simulink model "s0505_rollsensorfusion_EKF"  (R2021a)
settings: Solver=FixedStepAuto  StartTime=0.0  StopTime=10.0  RelTol=1e-3  EnableMultiTasking=on
undefined symbols (not defined in the file): Ts
libraries: CarMaker4SL x13, dspfdesign x2, dspmathops x2, sharedTrackingLibrary x1
settings Model: Creator=jason  LastModifiedBy=jason
settings ModelReferenceCC: ModelReferenceNumInstancesAllowed=Single

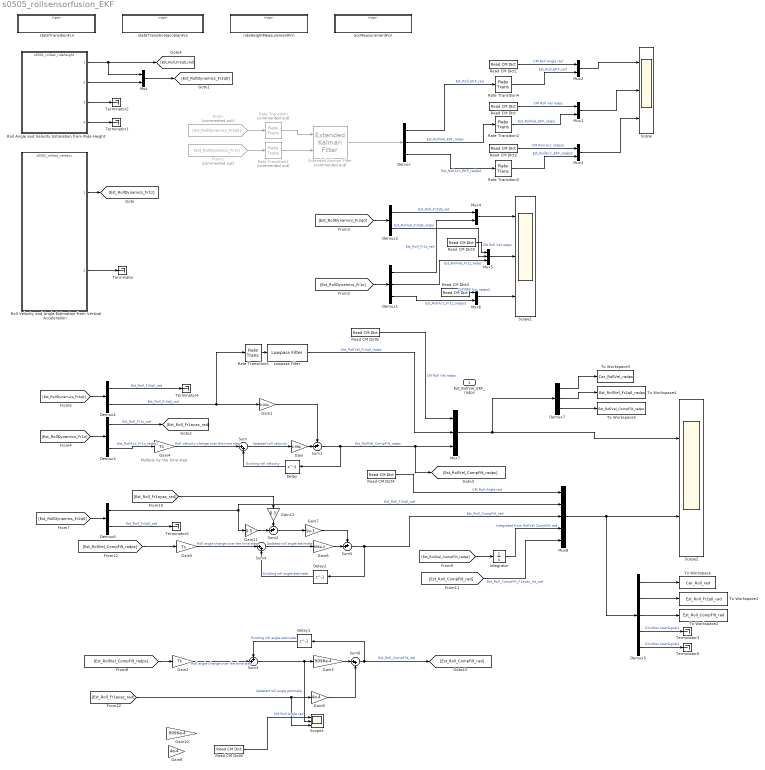
== system s0505_rollsensorfusion_EKF ==
  note: Multiply by the time step
  Delay : Delay  DelayLength=1
  Delay1 : Delay  DelayLength=1
  Delay2 : Delay  DelayLength=1
  Demux{,1,3,7} (4 alike) : Demux  Outputs=3
      Demux settings: DisplayOption=none
      Demux1 settings: DisplayOption=none
      Demux3 settings: DisplayOption=none
  Demux2 : Demux  Outputs=2
      settings: DisplayOption=none
  Demux4 : Demux  Outputs=2
      settings: DisplayOption=none
  Demux5 : Demux  Outputs=5
      settings: DisplayOption=none
  Demux6 : Demux  Outputs=2
      settings: DisplayOption=none
  Extended Kalman Filter : sharedTrackingLibrary/Extended Kalman Filter  Commented=on  StateTransitionFcn=stateTransitionFcn  HasStateTransitionJacobianFcn=off  StateTransitionJacobianFcn=stateTransitionJacobianFcn  HasAdditiveProcessNoise=Nonadditive  ProcessNoise=[0 0;0 0]  HasTimeVaryingProcessNoise=off  HasStateTransitionFcnExtraArgument=0  InitialState=[0; 0; 0]  InitialStateCovariance=1  MeasurementFcn1=rideHeightMeasurementFcn  HasMeasurementJacobianFcn1=off  HasMeasurementEnablePort1=off  HasAdditiveMeasurementNoise1=Nonadditive  MeasurementNoise1=[0.05^2 0; 0 0.05^2]  HasTimeVaryingMeasurementNoise1=off  HasMeasurementFcnExtraArgument1=0  MeasurementFcn2=accMeasurementFcn  HasMeasurementJacobianFcn2=off  HasMeasurementEnablePort2=off  HasAdditiveMeasurementNoise2=Nonadditive  MeasurementNoise2=0.05^2  HasTimeVaryingMeasurementNoise2=off  HasMeasurementFcnExtraArgument2=0  MeasurementFcn3=myMeasurementFcn  HasMeasurementJacobianFcn3=off  HasMeasurementEnablePort3=off  HasAdditiveMeasurementNoise3=Additive  MeasurementNoise3=1  HasTimeVaryingMeasurementNoise3=off  HasMeasurementFcnExtraArgument3=0  MeasurementFcn4=myMeasurementFcn  HasMeasurementJacobianFcn4=off  HasMeasurementEnablePort4=off  HasAdditiveMeasurementNoise4=Additive  MeasurementNoise4=1  HasTimeVaryingMeasurementNoise4=off  HasMeasurementFcnExtraArgument4=0  MeasurementFcn5=myMeasurementFcn  HasMeasurementJacobianFcn5=off  HasMeasurementEnablePort5=off  HasAdditiveMeasurementNoise5=Additive  MeasurementNoise5=1  HasTimeVaryingMeasurementNoise5=off  HasMeasurementFcnExtraArgument5=0  EnableMultirate=off  StateTransitionFcnSampleTime=1  MeasurementFcn1SampleTime=1  MeasurementFcn2SampleTime=1  MeasurementFcn3SampleTime=1  MeasurementFcn4SampleTime=1  MeasurementFcn5SampleTime=1  UseCurrentEstimator=on  OutputStateCovariance=off  DataType=double  SampleTime=1  NumberOfMeasurements=2
      settings: SourceProductBaseCode=CT,DR,TF,ID,LP,NV,AR,RO,RR,UV,VE
  From : From  Commented=on  GotoTag=Est_RollDynamics_Fr2q0
  From1 : From  Commented=on  GotoTag=Est_RollDynamics_Fr1z
  Gain : Gain  Gain=0.996
  Gain1 : Gain  Gain=0.004
  Gain10 : Gain  Gain=9996e-4
  Gain11 : Gain  Gain=0.5
  Gain12 : Gain  Gain=0.5
  Gain2 : Gain  Gain=Ts
  Gain3 : Gain  Gain=9996e-4
  Gain4 : Gain  Gain=Ts
  Gain5 : Gain  Gain=Ts
  Gain6 : Gain  Gain=995e-3
  Gain7 : Gain  Gain=5e-3
  Gain8 : Gain  Gain=4e-4
  Gain9 : Gain  Gain=4e-4
  Integrator : Integrator
  Lowpass Filter : dspfdesign/Lowpass Filter  FilterType=FIR  DesignForMinimumOrder=on  FilterOrder=50  PassbandFrequency=1  StopbandFrequency=2000  PassbandRipple=0.1  StopbandAttenuation=180  InheritSampleRate=off  SampleRate=44100  SimulateUsing=Interpreted execution  roundingMode=Floor  coeffsDataTypeStr=fixdt(1,16)
  Mux{,1..4,6} (6 alike) : Mux  Inputs=2
  Mux5 : Mux  Inputs=3
  Mux7 : Mux  Inputs=3
  Mux8 : Mux  Inputs=5
  Rate Transition : RateTransition  Commented=on
  Rate Transition1 : RateTransition  Commented=on
  Rate Transition{2..5} (4 alike) : RateTransition
  Read CM Dict : CarMaker4SL/Read CM Dict  xname=Car.RollVel  xsync=off  xstime=Continuous
  Read CM Dict1 : CarMaker4SL/Read CM Dict  xname=Car.Roll  xsync=off  xstime=Continuous
  Read CM Dict2 : CarMaker4SL/Read CM Dict  xname=Car.RollAcc  xsync=off  xstime=Continuous
  Read CM Dict3 : CarMaker4SL/Read CM Dict  xname=Car.RollAcc  xsync=off  xstime=Continuous
  Read CM Dict4 : CarMaker4SL/Read CM Dict  xname=Car.Roll  xsync=off  xstime=Continuous
  Read CM Dict5 : CarMaker4SL/Read CM Dict  xname=Car.RollVel  xsync=off  xstime=Continuous
  Read CM Dict6 : CarMaker4SL/Read CM Dict  xname=Car.RollVel  xsync=off  xstime=Continuous
  Read CM Dict8 : CarMaker4SL/Read CM Dict  xname=Car.Roll  xsync=off  xstime=Continuous
  Roll Angle and Velocity Estimation from Ride Height : ModelReference  ModelNameDialog=s0501_rollest_rideheight.slx  SimulationMode=Normal  ModelReferenceVersion=1.15
  Roll Velocity and Angle Estimation from Vertical Acceleration : ModelReference  ModelNameDialog=s0502_rollest_vertacc.slx  SimulationMode=Normal  ModelReferenceVersion=1.16
  Scope : Scope  NumInputPorts=3
  Scope1 : Scope  NumInputPorts=3
  Scope2 : Scope  NumInputPorts=2
  Scope4 : Scope  NumInputPorts=3
  Sum : Sum  Inputs=|++
  Sum{1..3,5} (4 alike) : Sum  Inputs=++|
  Sum4 : Sum  Inputs=|++
  Sum6 : Sum  Inputs=|++
  Terminator{,1..6} (7 alike) : Terminator
  To Workspace : ToWorkspace  VariableName=Car_Roll_rad  SampleTime=-1
  To Workspace1 : ToWorkspace  VariableName=Est_Roll_Fr2q0_rad  SampleTime=-1
  To Workspace2 : ToWorkspace  VariableName=Est_Roll_CompFilt_rad  SampleTime=-1
  To Workspace3 : ToWorkspace  VariableName=Car_RollVel_radps  SampleTime=-1
  To Workspace4 : ToWorkspace  VariableName=Est_RollVel_Fr2q0_radps  SampleTime=-1
  To Workspace5 : ToWorkspace  VariableName=Est_RollVel_CompFilt_radps  SampleTime=-1
  accMeasurementFcn : Subsystem  TreatAsAtomicUnit=on
  rideHeightMeasurementFcn : Subsystem  TreatAsAtomicUnit=on
  stateTransitionFcn : Subsystem  TreatAsAtomicUnit=on
  stateTransitionJacobianFcn : Subsystem  TreatAsAtomicUnit=on
  Est_RollVel_EKF_radps : Outport
  wires:
  Roll Angle and Velocity Estimation from Ride Height/2 -> Mux/2
  Extended Kalman Filter/1 -> Demux/1
  Roll Velocity and Angle Estimation from Vertical Acceleration/1 -> [Est_RollDynamics_Fr1z]
  Read CM Dict/1 -> Mux1/1  "CM Roll Vel radps"
  Roll Angle and Velocity Estimation from Ride Height/1 -> [Est_Roll_Fr2q0_rad], Mux/1
  Roll Velocity and Angle Estimation from Vertical Acceleration/2 -> Terminator/1
  Roll Angle and Velocity Estimation from Ride Height/4 -> Terminator1/1
  Roll Angle and Velocity Estimation from Ride Height/3 -> Terminator2/1
  Rate Transition/1 -> Extended Kalman Filter/1
  Rate Transition1/1 -> Extended Kalman Filter/2
  Mux1/1 -> Scope/2
  Demux/2 -> Rate Transition2/1  "Est_RollVel_EKF_radps"
  Mux2/1 -> Scope/1
  Read CM Dict1/1 -> Mux2/1  "CM Roll Angle rad"
  Demux/3 -> Rate Transition3/1  "Est_RollAcc_EKF_radps2"
  Rate Transition2/1 -> Mux1/2  "Est_RollVel_EKF_radps"
  Rate Transition3/1 -> Mux3/2  "Est_RollAcc_EKF_radps2"
  Demux/1 -> Rate Transition4/1  "Est_Roll_EKF_rad"
  Rate Transition4/1 -> Mux2/2  "Est_Roll_EKF_rad"
  Read CM Dict2/1 -> Mux3/1  "CM Roll Acc radps2"
  Mux3/1 -> Scope/3
  Mux4/1 -> Scope1/1
  Mux5/1 -> Scope1/2
  Mux6/1 -> Scope1/3
  Demux1/1 -> Mux4/2  "Est_Roll_Fr1z_rad"
  Demux1/2 -> Mux5/3  "Est_RollVel_Fr1z_radps"
  Demux1/3 -> Mux6/2  "Est_RollAcc_Fr1z_radps2"
  Read CM Dict3/1 -> Mux6/1  "CM Roll Acc radps2"
  Read CM Dict5/1 -> Mux5/1  "CM Roll Vel radps"
  Mux/1 -> [Est_RollDynamics_Fr2q0]
  From/1 -> Rate Transition/1
  From1/1 -> Rate Transition1/1
  [Est_RollDynamics_Fr1z] -> Demux1/1
  [Est_RollDynamics_Fr2q0] -> Demux2/1
  Demux2/1 -> Mux4/1  "Est_Roll_Fr2q0_rad"
  Demux2/2 -> Mux5/2  "Est_RollVel_Fr2q0_radps"
  [Est_RollDynamics_Fr2q0] -> Demux4/1
  [Est_RollDynamics_Fr1z] -> Demux3/1
  Sum/1 -> Gain/1  "Updated roll velocity"
  Delay/1 -> Sum/2  "Existing roll velocity"
  Gain/1 -> Sum1/2
  Gain1/1 -> Sum1/1
  Sum1/1 -> Delay/1, Mux7/3, [Est_RollVel_CompFilt_radps]  "Est_RollVel_CompFilt_radps"
  Demux4/2 -> Rate Transition5/1, Gain1/1  "Est_Roll_Fr2q0_rad"
  Demux3/3 -> Gain4/1  "Est_RollAcc_Fr1z_radps2"
  Read CM Dict6/1 -> Mux7/1  "CM Roll Vel radps"
  Mux7/1 -> Scope2/1, Demux7/1
  Gain4/1 -> Sum/1  "Roll velocity change over the time step"
  Lowpass Filter/1 -> Mux7/2  "Est_RollVel_Fr2q0_radps"
  Rate Transition5/1 -> Lowpass Filter/1
  Demux3/1 -> [Est_Roll_Fr1ayaz_rad]  "Est_Roll_Fr1z_rad"
  Gain5/1 -> Sum4/1  "Roll angle change over the time step"
  Sum5/1 -> Mux8/3, Delay2/1  "Est_Roll_CompFilt_rad"
  Delay2/1 -> Sum4/2  "Existing roll angle estimate"
  Gain6/1 -> Sum5/2
  Sum4/1 -> Gain6/1  "Updated roll angle estimate"
  [Est_RollDynamics_Fr2q0] -> Demux6/1
  Demux6/1 -> Gain11/1, Mux8/2  "Est_Roll_Fr2q0_rad"
  Gain7/1 -> Sum5/1
  Demux4/1 -> Terminator4/1  "Est_Roll_Fr2q0_rad"
  Demux6/2 -> Terminator5/1  "Est_Roll_Fr2q0_rad"
  Mux8/1 -> Demux5/1, Scope2/2
  Read CM Dict4/1 -> Mux8/1  "CM Roll Angle rad"
  [Est_RollVel_CompFilt_radps] -> Gain5/1
  Sum3/1 -> Scope4/2, Gain3/1  "Updated roll angle estimate"
  Gain2/1 -> Sum3/2  "Roll angle change over the time step"
  Delay1/1 -> Sum3/1  "Existing roll angle estimate"
  Sum6/1 -> Delay1/1, [Est_Roll_CompFilt_rad]  "Est_Roll_CompFilt_rad"
  [Est_Roll_Fr1ayaz_rad] -> Scope4/3, Gain8/1
  Gain8/1 -> Sum6/2
  Gain3/1 -> Sum6/1
  [Est_RollVel_CompFilt_radps] -> Gain2/1
  Read CM Dict8/1 -> Scope4/1  "CM Roll Angle rad"
  [Est_RollVel_CompFilt_radps] -> Integrator/1
  Integrator/1 -> Mux8/4  "Integrated from RollVel CompFilt rad"
  [Est_Roll_CompFilt_rad] -> Mux8/5  "Est_Roll_CompFilt_F1ayaz_Int_rad"
  [Est_Roll_Fr1ayaz_rad] -> Gain12/1
  Gain11/1 -> Sum2/2
  Gain12/1 -> Sum2/1
  Sum2/1 -> Gain7/1
  Demux5/1 -> To Workspace/1
  Demux5/2 -> To Workspace1/1
  Demux5/3 -> To Workspace2/1
  Demux5/4 -> Terminator3/1  "DrivMan UserSignal1"
  Demux5/5 -> Terminator6/1  "DrivMan UserSignal2"
  Demux7/1 -> To Workspace3/1
  Demux7/2 -> To Workspace4/1
  Demux7/3 -> To Workspace5/1

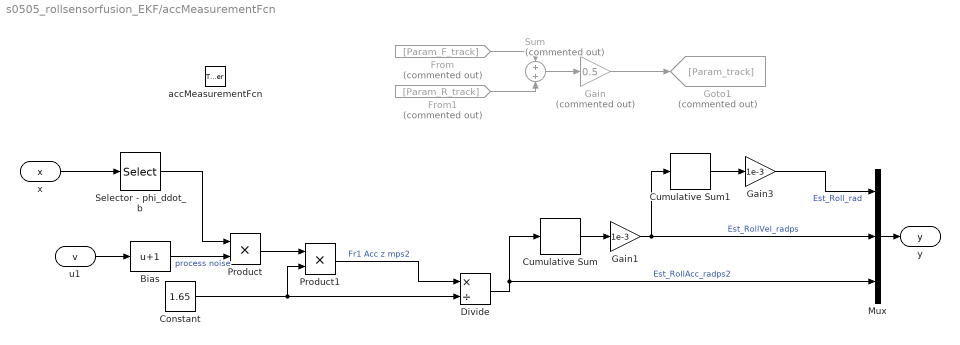
== system s0505_rollsensorfusion_EKF/accMeasurementFcn ==
  accMeasurementFcn : TriggerPort  TriggerType=function-call  IsSimulinkFunction=on  FunctionName=accMeasurementFcn  FunctionVisibility=scoped  VariantControl=(inherit)
  Bias : Bias  Bias=1
  Constant : Constant  Value=1.65
  Cumulative Sum : dspmathops/Cumulative Sum  dim=Channels (running sum)  InputProcessing=Columns as channels (frame based)  reset_popup=None  roundingMode=Floor  overflowMode=off  outputDataTypeStr=Inherit: Same as accumulator  outputMin=[]  outputMax=[]  outputLastDataTypeStr=Inherit: Same as accumulator
  Cumulative Sum1 : dspmathops/Cumulative Sum  dim=Channels (running sum)  InputProcessing=Columns as channels (frame based)  reset_popup=None  roundingMode=Floor  overflowMode=off  outputDataTypeStr=Inherit: Same as accumulator  outputMin=[]  outputMax=[]  outputLastDataTypeStr=Inherit: Same as accumulator
  Divide : Product  Inputs=*/
  From : From  Commented=on  GotoTag=Param_F_track
  From1 : From  Commented=on  GotoTag=Param_R_track
  Gain : Gain  Commented=on  Gain=0.5
  Gain1 : Gain  Gain=1e-3
  Gain3 : Gain  Gain=1e-3
  Goto1 : Goto  Commented=on  GotoTag=Param_track
  Mux : Mux  Inputs=3
  Product : Product
  Product1 : Product
  Selector - phi_ddot_b : Selector  InputPortWidth=3  IndexOptions=Index vector (dialog)  Indices=[3]  OutputSizes=1
  Sum : Sum  Commented=on  Inputs=+|+
  x : ArgIn  DisableCoverage=on  PortDimensions=3  ArgumentName=x
  u1 : ArgIn  DisableCoverage=on  Port=2  ArgumentName=v
  y : ArgOut  DisableCoverage=on  PortDimensions=3  ArgumentName=y
  wires:
  x/1 -> Selector - phi_ddot_b/1
  From/1 -> Sum/1
  From1/1 -> Sum/2
  Sum/1 -> Gain/1
  Gain/1 -> Goto1/1
  Mux/1 -> y/1
  Divide/1 -> Cumulative Sum/1, Mux/3  "Est_RollAcc_radps2"
  Selector - phi_ddot_b/1 -> Product/1
  Constant/1 -> Divide/2, Product1/2
  Product1/1 -> Divide/1  "Fr1 Acc z mps2"
  Bias/1 -> Product/2  "process noise"
  u1/1 -> Bias/1
  Product/1 -> Product1/1
  Gain1/1 -> Cumulative Sum1/1, Mux/2  "Est_RollVel_radps"
  Gain3/1 -> Mux/1  "Est_Roll_rad"
  Cumulative Sum/1 -> Gain1/1
  Cumulative Sum1/1 -> Gain3/1

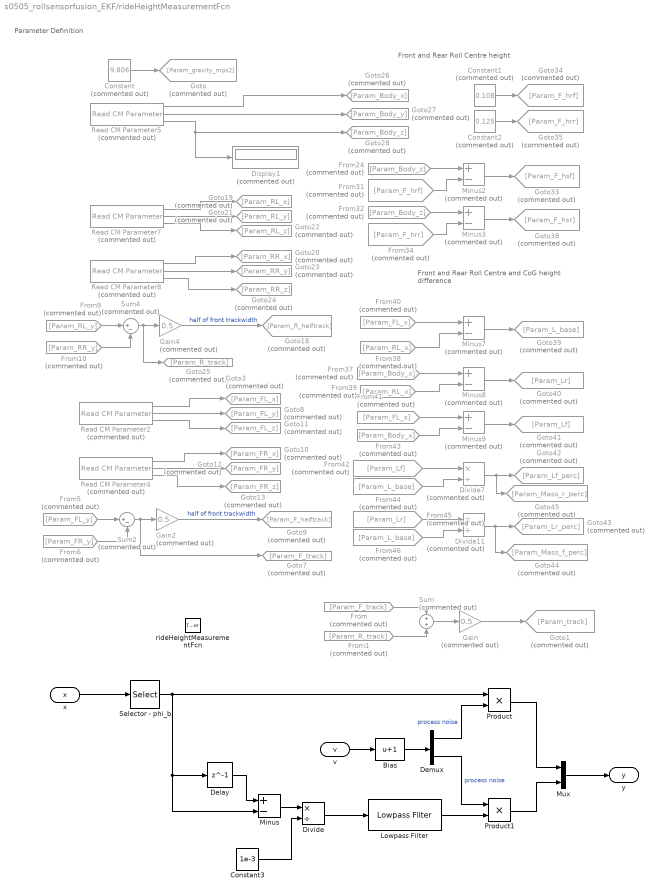
== system s0505_rollsensorfusion_EKF/rideHeightMeasurementFcn ==
  note: Parameter Definition
  note: Front and Rear Roll Centre height
  note: Front and Rear Roll Centre and CoG height difference
  rideHeightMeasurementFcn : TriggerPort  TriggerType=function-call  IsSimulinkFunction=on  FunctionName=rideHeightMeasurementFcn  FunctionVisibility=scoped  VariantControl=(inherit)
  Bias : Bias  Bias=1
  Constant : Constant  Commented=on  Value=9.806
  Constant1 : Constant  Commented=on  Value=0.108
  Constant2 : Constant  Commented=on  Value=0.125
  Constant3 : Constant  Value=1e-3
  Delay : Delay  DelayLength=1
  Demux : Demux  Outputs=2
      settings: DisplayOption=none
  Display1 : Display  Commented=on
  Divide : Product  Inputs=*/
  Divide11 : Product  Commented=on  Inputs=*/
  Divide7 : Product  Commented=on  Inputs=*/
  From : From  Commented=on  GotoTag=Param_F_track
  From1 : From  Commented=on  GotoTag=Param_R_track
  From10 : From  Commented=on  GotoTag=Param_RR_y
  From24 : From  Commented=on  GotoTag=Param_Body_z
  From31 : From  Commented=on  GotoTag=Param_F_hrf
  From32 : From  Commented=on  GotoTag=Param_Body_z
  From34 : From  Commented=on  GotoTag=Param_F_hrr
  From37 : From  Commented=on  GotoTag=Param_Body_x
  From38 : From  Commented=on  GotoTag=Param_RL_x
  From39 : From  Commented=on  GotoTag=Param_RL_x
  From40 : From  Commented=on  GotoTag=Param_FL_x
  From41 : From  Commented=on  GotoTag=Param_FL_x
  From42 : From  Commented=on  GotoTag=Param_Lf
  From43 : From  Commented=on  GotoTag=Param_Body_x
  From44 : From  Commented=on  GotoTag=Param_L_base
  From45 : From  Commented=on  GotoTag=Param_Lr
  From46 : From  Commented=on  GotoTag=Param_L_base
  From5 : From  Commented=on  GotoTag=Param_FL_y
  From6 : From  Commented=on  GotoTag=Param_FR_y
  From9 : From  Commented=on  GotoTag=Param_RL_y
  Gain : Gain  Commented=on  Gain=0.5
  Gain2 : Gain  Commented=on  Gain=0.5
  Gain4 : Gain  Commented=on  Gain=0.5
  Goto : Goto  Commented=on  GotoTag=Param_gravity_mps2
  Goto1 : Goto  Commented=on  GotoTag=Param_track
  Goto10 : Goto  Commented=on  GotoTag=Param_FR_x
  Goto11 : Goto  Commented=on  GotoTag=Param_FL_z
  Goto12 : Goto  Commented=on  GotoTag=Param_FR_y
  Goto13 : Goto  Commented=on  GotoTag=Param_FR_z
  Goto18 : Goto  Commented=on  GotoTag=Param_R_halftrack
  Goto19 : Goto  Commented=on  GotoTag=Param_RL_x
  Goto20 : Goto  Commented=on  GotoTag=Param_RR_x
  Goto21 : Goto  Commented=on  GotoTag=Param_RL_y
  Goto22 : Goto  Commented=on  GotoTag=Param_RL_z
  Goto23 : Goto  Commented=on  GotoTag=Param_RR_y
  Goto24 : Goto  Commented=on  GotoTag=Param_RR_z
  Goto25 : Goto  Commented=on  GotoTag=Param_R_track
  Goto26 : Goto  Commented=on  GotoTag=Param_Body_x
  Goto27 : Goto  Commented=on  GotoTag=Param_Body_y
  Goto28 : Goto  Commented=on  GotoTag=Param_Body_z
  Goto3 : Goto  Commented=on  GotoTag=Param_FL_x
  Goto33 : Goto  Commented=on  GotoTag=Param_F_hsf
  Goto34 : Goto  Commented=on  GotoTag=Param_F_hrf
  Goto35 : Goto  Commented=on  GotoTag=Param_F_hrr
  Goto38 : Goto  Commented=on  GotoTag=Param_F_hsr
  Goto39 : Goto  Commented=on  GotoTag=Param_L_base
  Goto40 : Goto  Commented=on  GotoTag=Param_Lr
  Goto41 : Goto  Commented=on  GotoTag=Param_Lf
  Goto42 : Goto  Commented=on  GotoTag=Param_Lf_perc
  Goto43 : Goto  Commented=on  GotoTag=Param_Lr_perc
  Goto44 : Goto  Commented=on  GotoTag=Param_Mass_f_perc
  Goto45 : Goto  Commented=on  GotoTag=Param_Mass_r_perc
  Goto7 : Goto  Commented=on  GotoTag=Param_F_track
  Goto8 : Goto  Commented=on  GotoTag=Param_FL_y
  Goto9 : Goto  Commented=on  GotoTag=Param_F_halftrack
  Lowpass Filter : dspfdesign/Lowpass Filter  FilterType=FIR  DesignForMinimumOrder=on  FilterOrder=50  PassbandFrequency=1  StopbandFrequency=2000  PassbandRipple=0.1  StopbandAttenuation=180  InheritSampleRate=off  SampleRate=44100  SimulateUsing=Interpreted execution  roundingMode=Floor  coeffsDataTypeStr=fixdt(1,16)
  Minus : Sum  Inputs=+-
  Minus{2..3,7..9} (5 alike) : Sum  Commented=on  Inputs=+-
  Mux : Mux  Inputs=2
  Product : Product
  Product1 : Product
  Read CM Parameter2 : CarMaker4SL/Read CM Parameter  Commented=on  xfile=Vehicle  xkey=WheelCarrier.fl.pos  xnout=3  xdefaults=eps  xmuxed=off  xstime=Continuous
      settings: SourceProductName=CarMaker4SL
  Read CM Parameter4 : CarMaker4SL/Read CM Parameter  Commented=on  xfile=Vehicle  xkey=WheelCarrier.fr.pos  xnout=3  xdefaults=eps  xmuxed=off  xstime=Continuous
      settings: SourceProductName=CarMaker4SL
  Read CM Parameter5 : CarMaker4SL/Read CM Parameter  Commented=on  xfile=Vehicle  xkey=Body.pos  xnout=3  xdefaults=eps  xmuxed=off  xstime=Continuous
      settings: SourceProductName=CarMaker4SL
  Read CM Parameter7 : CarMaker4SL/Read CM Parameter  Commented=on  xfile=Vehicle  xkey=WheelCarrier.rl.pos  xnout=3  xdefaults=eps  xmuxed=off  xstime=Continuous
      settings: SourceProductName=CarMaker4SL
  Read CM Parameter8 : CarMaker4SL/Read CM Parameter  Commented=on  xfile=Vehicle  xkey=WheelCarrier.rr.pos  xnout=3  xdefaults=eps  xmuxed=off  xstime=Continuous
      settings: SourceProductName=CarMaker4SL
  Selector - phi_b : Selector  InputPortWidth=3  IndexOptions=Index vector (dialog)  Indices=[1]  OutputSizes=1
  Sum : Sum  Commented=on  Inputs=+|+
  Sum2 : Sum  Commented=on  Inputs=|+-
  Sum4 : Sum  Commented=on  Inputs=|+-
  x : ArgIn  DisableCoverage=on  PortDimensions=3  ArgumentName=x
  v : ArgIn  DisableCoverage=on  Port=2  PortDimensions=2  ArgumentName=v
  y : ArgOut  DisableCoverage=on  PortDimensions=2  ArgumentName=y
  wires:
  x/1 -> Selector - phi_b/1
  Sum2/1 -> Gain2/1, Goto7/1
  Divide11/1 -> Goto44/1, Goto43/1
  From46/1 -> Divide11/2
  From45/1 -> Divide11/1
  Minus7/1 -> Goto39/1
  From40/1 -> Minus7/1
  From42/1 -> Divide7/1
  Read CM Parameter7/1 -> Goto19/1
  From9/1 -> Sum4/1
  From32/1 -> Minus3/1
  Constant2/1 -> Goto35/1
  Read CM Parameter2/3 -> Goto11/1
  From37/1 -> Minus8/1
  From24/1 -> Minus2/1
  Constant1/1 -> Goto34/1
  Read CM Parameter8/1 -> Goto20/1
  Read CM Parameter4/1 -> Goto10/1
  Read CM Parameter8/2 -> Goto23/1
  Divide7/1 -> Goto45/1, Goto42/1
  Read CM Parameter5/1 -> Goto26/1
  From6/1 -> Sum2/2
  Read CM Parameter7/3 -> Goto22/1
  Read CM Parameter5/2 -> Goto27/1
  Constant/1 -> Goto/1
  From10/1 -> Sum4/2
  From31/1 -> Minus2/2
  Minus2/1 -> Goto33/1
  Minus8/1 -> Goto40/1
  Read CM Parameter2/2 -> Goto8/1
  Gain2/1 -> Goto9/1  "half of front trackwidth"
  Minus3/1 -> Goto38/1
  Sum4/1 -> Gain4/1, Goto25/1
  From39/1 -> Minus8/2
  From38/1 -> Minus7/2
  Read CM Parameter5/3 -> Display1/1, Goto28/1
  Read CM Parameter7/2 -> Goto21/1
  From34/1 -> Minus3/2
  From5/1 -> Sum2/1
  Minus9/1 -> Goto41/1
  From43/1 -> Minus9/2
  From41/1 -> Minus9/1
  Read CM Parameter4/2 -> Goto12/1
  Read CM Parameter2/1 -> Goto3/1
  Read CM Parameter4/3 -> Goto13/1
  Read CM Parameter8/3 -> Goto24/1
  Gain4/1 -> Goto18/1  "half of front trackwidth"
  From44/1 -> Divide7/2
  From/1 -> Sum/1
  From1/1 -> Sum/2
  Sum/1 -> Gain/1
  Gain/1 -> Goto1/1
  v/1 -> Bias/1
  Mux/1 -> y/1
  Bias/1 -> Demux/1
  Demux/1 -> Product/2  "process noise"
  Lowpass Filter/1 -> Product1/2
  Demux/2 -> Product1/1  "process noise"
  Product1/1 -> Mux/2
  Product/1 -> Mux/1
  Selector - phi_b/1 -> Delay/1, Minus/2, Product/1
  Delay/1 -> Minus/1
  Minus/1 -> Divide/1
  Constant3/1 -> Divide/2
  Divide/1 -> Lowpass Filter/1

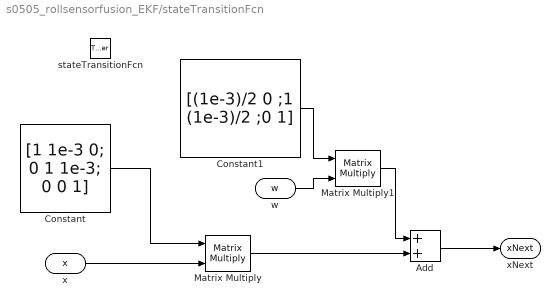
== system s0505_rollsensorfusion_EKF/stateTransitionFcn ==
  stateTransitionFcn : TriggerPort  TriggerType=function-call  IsSimulinkFunction=on  FunctionName=stateTransitionFcn  FunctionVisibility=scoped  VariantControl=(inherit)
  Add : Sum
  Constant : Constant  Value=[1 1e-3 0; 0 1 1e-3; 0 0 1]
  Constant1 : Constant  Value=[(1e-3)/2 0 ;1 (1e-3)/2 ;0 1]  VectorParams1D=off
  Matrix Multiply : Product  Multiplication=Matrix(*)
  Matrix Multiply1 : Product  Multiplication=Matrix(*)
  x : ArgIn  DisableCoverage=on  PortDimensions=3  ArgumentName=x
  w : ArgIn  DisableCoverage=on  Port=2  PortDimensions=2  ArgumentName=w
  xNext : ArgOut  DisableCoverage=on  PortDimensions=3  ArgumentName=xNext
  wires:
  Constant1/1 -> Matrix Multiply1/1
  w/1 -> Matrix Multiply1/2
  Add/1 -> xNext/1
  Matrix Multiply1/1 -> Add/1
  Matrix Multiply/1 -> Add/2
  x/1 -> Matrix Multiply/2
  Constant/1 -> Matrix Multiply/1

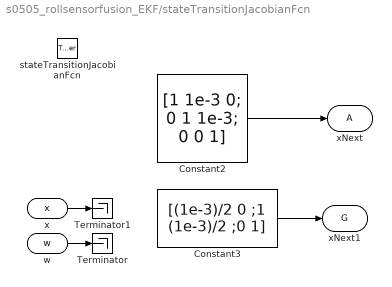
== system s0505_rollsensorfusion_EKF/stateTransitionJacobianFcn ==
  stateTransitionJacobianFcn : TriggerPort  TriggerType=function-call  IsSimulinkFunction=on  FunctionName=stateTransitionJacobianFcn  FunctionVisibility=scoped  VariantControl=(inherit)
  Constant2 : Constant  Value=[1 1e-3 0; 0 1 1e-3; 0 0 1]
  Constant3 : Constant  Value="[(1e-3)/2 0  ;1 (1e-3)/2 ;0 1]"
  Terminator : Terminator
  Terminator1 : Terminator
  x : ArgIn  DisableCoverage=on  PortDimensions=3  ArgumentName=x
  w : ArgIn  DisableCoverage=on  Port=2  PortDimensions=3  ArgumentName=w
  xNext : ArgOut  DisableCoverage=on  PortDimensions=[3 3]  ArgumentName=A
  xNext1 : ArgOut  DisableCoverage=on  Port=2  PortDimensions=[3 2]  ArgumentName=G
  wires:
  Constant2/1 -> xNext/1
  w/1 -> Terminator/1
  x/1 -> Terminator1/1
  Constant3/1 -> xNext1/1
